simulink model "VAD"  (R2020a)
settings: Solver=VariableStepAuto  StartTime=0.0  StopTime=15  RelTol=1e-3
libraries: dspvision x1, dspstat3 x1
settings Model: Creator=Michele  LastModifiedBy=miche
settings DataIOCC: ReturnWorkspaceOutputs=off
settings DebuggingCC: ArithmeticOperatorsInVariantConditions=warning
settings SFSimCC: SimUseLocalCustomCode=off  CustomCodeUndefinedFunction=UseInterfaceOnly
settings RTWCC: RTWUseLocalCustomCode=off
settings CodeAppCC: StateflowObjectComments=on

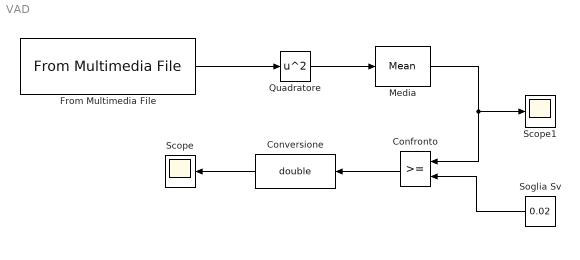
== system VAD ==
  Confronto : RelationalOperator  OutDataTypeStr=boolean  RndMeth=Simplest
  Conversione : DataTypeConversion  OutDataTypeStr=double  RndMeth=Nearest
  From Multimedia File : dspvision/From Multimedia File  inputFilename=C:\Program Files\MATLAB\R2020a\toolbox\audio\samples\Counting-16-44p1-mono-15secs.wav  readRange=[1 Inf]  loop=on  numPlays=inf  outputStreams=Audio only  videoDataType=single  audioDataType=double  inheritSampleTime=on  userDefinedSampleTime=1/30  noAudioOutput=off  isIntensityVideo=off  fourcc=RGB  colorVideoFormat=Separate color signals  outputEOF=off  dataOrg=Column-major  audioFrameSize=4096  computeAudioFrameSize=off  outSamplingMode=Sample based
  Media : dspstat3/Mean  run=off  reset_popup=None  directionMode=Each column  dimension=1  roiEnable=off  roiType=Rectangles  roiPortion=Entire ROI  roiOutput=Individual statistics for each ROI  roiFlag=off  roundingMode=Floor  overflowMode=off  outputDataTypeStr=Inherit: Same as accumulator  outputMin=[]  outputMax=[]  outputLastDataTypeStr=Inherit: Same as accumulator
  Quadratore : Math  Operator=square  SignedPower=on  SaturateOnIntegerOverflow=on
  Scope : Scope
  Scope1 : Scope
  "Soglia Sv " : Constant  Value=0.02
  wires:
  From Multimedia File/1 -> Quadratore/1
  Quadratore/1 -> Media/1
  Confronto/1 -> Conversione/1
  Conversione/1 -> Scope/1
  Media/1 -> Scope1/1, Confronto/1
  "Soglia Sv "/1 -> Confronto/2
